simulink model "Example_3"  (R2020b)
settings: Solver=VariableStepAuto  StartTime=0.0  StopTime=10.0  RelTol=1e-3
libraries: fl_lib x17, nesl_utility x6
settings Model: Creator=zaliyazici  LastModifiedBy=zaliyazici

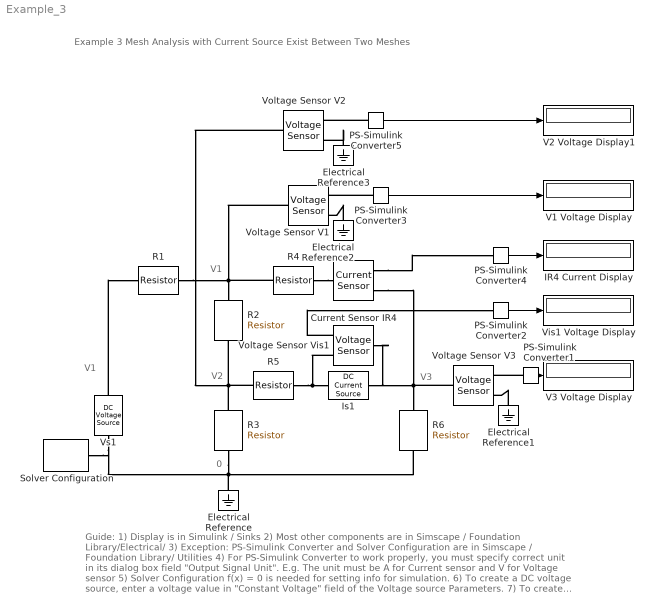
== system Example_3 ==
  note: V1
  note: V1
  note: V3
  note: Example 3 Mesh Analysis with Current Source Exist Between Two Meshes
  note: Guide:
      | 1) Display is in Simulink / Sinks
      | 2) Most other components are in Simscape / Foundation Library/Electrical/
      | 3) Exception: PS-Simulink Converter and Solver Configuration are in Simscape / Foundation Library/ Utilities
      | 4) For PS-Simulink Converter to work properly, you must specify correct unit in its dialog box field "Output Signal Unit".
      | E.g. The unit must be A for Current sensor and V for Voltage sensor
      | 5) Solver Configuration f(x) = 0 is needed for setting info for simulation.
      | 6) To create a DC voltage source, enter a voltage value in "Constant Voltage" field of the Voltage source Parameters.
      | 7) To create "Annotation", double-click a location on project page and select "Create annotation" from the prompt. Then, type any text you want to clarify your circuit. E.g. "Display for Current".
      | 8) To understand how to use a component, right-click on the component and select "Help".
      | Measurement: Node voltages V1, V2, V3, voltage cross current source Is1, and current through R4
  note: 0
  note: V2
  Current Sensor IR4 : fl_lib/Electrical/Electrical Sensors/Current Sensor
  Electrical Reference{,1..3} (4 alike) : fl_lib/Electrical/Electrical Elements/Electrical Reference
  "IR4 Current Display " : Display
  Is1 : fl_lib/Electrical/Electrical Sources/DC Current Source  i0=4 mA
      settings: AttributesFormatString=%<i0> %<i0_unit>  SourceProductBaseCode=SS  InternalSimscapePortConfiguration="{\"Bottom\":[],\"Left\":[{\"id\":\"p\",\"label\":\"\",\"type\":\"foundation.electrical.electrical\"}],\"Right\":[{\"id\":\"n\",\"label\":\"\",\"type\":\"foundation.electrical.electrical\"}],\"Top\":[]}"
  PS-Simulink Converter{1..3,5} (4 alike) : nesl_utility/PS-Simulink Converter  PhysicalDomain=network_engine_domain  SubClassName=ps_output  LeftPortType=input  RightPortType=output  PseudoPeriodic=off  Frequencies=[]  Unit=V  AffineConversion=off
  PS-Simulink Converter4 : nesl_utility/PS-Simulink Converter  PhysicalDomain=network_engine_domain  SubClassName=ps_output  LeftPortType=input  RightPortType=output  PseudoPeriodic=off  Frequencies=[]  Unit=A  AffineConversion=off
  R1 : fl_lib/Electrical/Electrical Elements/Resistor  R=1 kOhm  i_specify=off  i_priority=None  i=0 A  i_nominal_specify=off  i_nominal_unit=A  i_nominal_value=1  v_specify=off  v_priority=None  v=0 V  v_nominal_specify=off  v_nominal_unit=V  v_nominal_value=1
      settings: AttributesFormatString=%<R> %<R_unit>  LogSimulationData=on
  R2 : fl_lib/Electrical/Electrical Elements/Resistor  R=1.2 kOhm  i_specify=off  i_priority=None  i=0 A  i_nominal_specify=off  i_nominal_unit=A  i_nominal_value=1  v_specify=off  v_priority=None  v=0 V  v_nominal_specify=off  v_nominal_unit=V  v_nominal_value=1
      settings: AttributesFormatString=%<R> %<R_unit>  LogSimulationData=on
  R3 : fl_lib/Electrical/Electrical Elements/Resistor  R=2 kOhm  i_specify=off  i_priority=None  i=0 A  i_nominal_specify=off  i_nominal_unit=A  i_nominal_value=1  v_specify=off  v_priority=None  v=0 V  v_nominal_specify=off  v_nominal_unit=V  v_nominal_value=1
      settings: AttributesFormatString=%<R> %<R_unit>  LogSimulationData=on
  R4 : fl_lib/Electrical/Electrical Elements/Resistor  R=4 kOhm  i_specify=off  i_priority=None  i=0 A  i_nominal_specify=off  i_nominal_unit=A  i_nominal_value=1  v_specify=off  v_priority=None  v=0 V  v_nominal_specify=off  v_nominal_unit=V  v_nominal_value=1
      settings: AttributesFormatString=%<R> %<R_unit>  LogSimulationData=on
  R5 : fl_lib/Electrical/Electrical Elements/Resistor  R=2 kOhm  i_specify=off  i_priority=None  i=0 A  i_nominal_specify=off  i_nominal_unit=A  i_nominal_value=1  v_specify=off  v_priority=None  v=0 V  v_nominal_specify=off  v_nominal_unit=V  v_nominal_value=1
      settings: AttributesFormatString=%<R> %<R_unit>  LogSimulationData=on
  R6 : fl_lib/Electrical/Electrical Elements/Resistor  R=800 Ohm  i_specify=off  i_priority=None  i=0 A  i_nominal_specify=off  i_nominal_unit=A  i_nominal_value=1  v_specify=off  v_priority=None  v=0 V  v_nominal_specify=off  v_nominal_unit=V  v_nominal_value=1
      settings: AttributesFormatString=%<R> %<R_unit>  LogSimulationData=on
  Solver Configuration : nesl_utility/Solver Configuration  PhysicalDomain=network_engine_domain  SubClassName=solver  LeftPortType=input  RightPortType=generic  Tones=[]  Harmonics=[]  SimulateNoise=off  Profile=off  UseLocalSampling=off  EnableSwitchedLinearOptims=on  FrequencyDomain=off  UseCCode=off  RelTol=0.001  AbsTol=1e-06  MinStep=1e-09  ToWorkspace=off  RevertToSquareIcSolve=off  NumHomotopyIterations=100  PhasorMode=off  PhasorModeNumHarmonics=1  DoDC=off  ResidualTolerance=1e-09  UseLocalSolver=off  LocalSolverChoice=NE_BACKWARD_EULER_ADVANCER  LocalSolverSampleTime=0.001  DoFixedCost=off  MaxNonlinIter=3  MaxModeIter=2  ComputeImpulses=off  ImpulseIterations=2  LinearAlgebra=auto  EquationFormulation=NE_TIME_EF  DelaysMemoryBudget=1024  AutomaticFiltering=on  FilteringTimeConstant=0.001  PartitionStorageMethod=AS_NEEDED  PartitionMemoryBudget=1024  PartitionMethod=ROBUST
  V1 Voltage Display : Display
  V2 Voltage Display1 : Display
  V3 Voltage Display : Display
  Vis1 Voltage Display : Display
  Voltage Sensor V1 : fl_lib/Electrical/Electrical Sensors/Voltage Sensor
  Voltage Sensor V2 : fl_lib/Electrical/Electrical Sensors/Voltage Sensor
  Voltage Sensor V3 : fl_lib/Electrical/Electrical Sensors/Voltage Sensor
  Voltage Sensor Vis1 : fl_lib/Electrical/Electrical Sensors/Voltage Sensor
  Vs1 : fl_lib/Electrical/Electrical Sources/DC Voltage Source  v0=10 V
      settings: AttributesFormatString=%<v0> %<v0_unit>
  wires:
  PS-Simulink Converter1/1 -> V3 Voltage Display/1
  PS-Simulink Converter4/1 -> "IR4 Current Display "/1
  PS-Simulink Converter3/1 -> V1 Voltage Display/1
  PS-Simulink Converter2/1 -> Vis1 Voltage Display/1
  PS-Simulink Converter5/1 -> V2 Voltage Display1/1
  connections:
  Vs1/LConn1 -- R1/LConn1
  R3/LConn1 -- R2/RConn1 -- Voltage Sensor V2/LConn1 -- R5/LConn1
  Vs1/RConn1 -- Solver Configuration/RConn1 -- R6/RConn1 -- R3/RConn1 -- Electrical Reference/LConn1
  Electrical Reference1/LConn1 -- Voltage Sensor V3/RConn2
  PS-Simulink Converter1/LConn1 -- Voltage Sensor V3/RConn1
  Voltage Sensor V3/LConn1 -- Current Sensor IR4/RConn2 -- Voltage Sensor Vis1/LConn1 -- Is1/LConn1 -- R6/LConn1
  Current Sensor IR4/RConn1 -- PS-Simulink Converter4/LConn1
  PS-Simulink Converter3/LConn1 -- Voltage Sensor V1/RConn1
  R1/RConn1 -- R2/LConn1 -- Voltage Sensor V1/LConn1 -- R4/LConn1
  R4/RConn1 -- Current Sensor IR4/LConn1
  Electrical Reference2/LConn1 -- Voltage Sensor V1/RConn2
  Voltage Sensor Vis1/RConn1 -- PS-Simulink Converter2/LConn1
  Voltage Sensor Vis1/RConn2 -- R5/RConn1 -- Is1/RConn1
  PS-Simulink Converter5/LConn1 -- Voltage Sensor V2/RConn1
  Electrical Reference3/LConn1 -- Voltage Sensor V2/RConn2
